simulink model "test_mdl1"  (R2023a)
settings: Solver=VariableStepAuto  StartTime=0.0  StopTime=10.0  RelTol=1e-3
(part 6 of 8)

== system test_mdl1/VehicleCAN/IPMA_ADAS/IPMA_Data3 ==
  AdbUrbanArea_B_Stat : Constant  Value=0
  CbdblActv_B_RqAdas : Constant  Value=0
  LightCurv_NoRate_Actl : Constant  Value=0
  LightCurv_No_Actl : Constant  Value=0
  LightPathOffst_L_Actl : Constant  Value=0
  LightPath_An_Actl : Constant  Value=0
  LightRng_L_Max : Constant  Value=0
  MbdblActv_B_RqAdas : Constant  Value=0
  bus_creator : BusCreator  Inputs=8
  out_port : Outport
  wires:
  bus_creator/1 -> out_port/1  "test_mdl1"
  AdbUrbanArea_B_Stat/1 -> bus_creator/1  "AdbUrbanArea_B_Stat"
  CbdblActv_B_RqAdas/1 -> bus_creator/2  "CbdblActv_B_RqAdas"
  LightCurv_NoRate_Actl/1 -> bus_creator/3  "LightCurv_NoRate_Actl"
  LightCurv_No_Actl/1 -> bus_creator/4  "LightCurv_No_Actl"
  LightPathOffst_L_Actl/1 -> bus_creator/5  "LightPathOffst_L_Actl"
  LightPath_An_Actl/1 -> bus_creator/6  "LightPath_An_Actl"
  LightRng_L_Max/1 -> bus_creator/7  "LightRng_L_Max"
  MbdblActv_B_RqAdas/1 -> bus_creator/8  "MbdblActv_B_RqAdas"

== system test_mdl1/VehicleCAN/IPMA_ADAS/IPMA_Data4 ==
  AdasLcDistToObj_L_Actl : Constant  Value=0
  VehVActlAdas_D_Qf : Constant  Value=0
  Veh_V_ActlAdas : Constant  Value=0
  Veh_V_RqLsc : Constant  Value=0
  bus_creator : BusCreator  Inputs=4
  out_port : Outport
  wires:
  bus_creator/1 -> out_port/1  "test_mdl1"
  AdasLcDistToObj_L_Actl/1 -> bus_creator/1  "AdasLcDistToObj_L_Actl"
  VehVActlAdas_D_Qf/1 -> bus_creator/2  "VehVActlAdas_D_Qf"
  Veh_V_ActlAdas/1 -> bus_creator/3  "Veh_V_ActlAdas"
  Veh_V_RqLsc/1 -> bus_creator/4  "Veh_V_RqLsc"

== system test_mdl1/VehicleCAN/IPMA_ADAS/Image_Processing_Data ==
  BrkDecel_B_RqRba : Constant  Value=0
  BrkEnbl_B_RqRba : Constant  Value=0
  CamraFrntStat_D_Stat : Constant  Value=0
  RbaAlrt_D_Dsply : Constant  Value=0
  RbaMnu_D_Rq : Constant  Value=0
  RbaMsg_D_Rq : Constant  Value=0
  Rba_D_Stat : Constant  Value=0
  TrlrAidEnbl_D_RqAdas : Constant  Value=0
  TrlrAidSwtchLamp_B_Rq : Constant  Value=0
  TrlrHitchChime_D_Rq : Constant  Value=0
  TrlrHitchIcon_D_Rq : Constant  Value=0
  TrlrHitchLamp_D_Rq2 : Constant  Value=0
  TrlrHitchMsgTxt_D_Rq : Constant  Value=0
  TrlrRvrseEnbl_D2_Stat : Constant  Value=0
  TrlrRvrseMsgTxt_D2_Rq : Constant  Value=0
  bus_creator : BusCreator  Inputs=15
  out_port : Outport
  wires:
  bus_creator/1 -> out_port/1  "test_mdl1"
  BrkDecel_B_RqRba/1 -> bus_creator/1  "BrkDecel_B_RqRba"
  BrkEnbl_B_RqRba/1 -> bus_creator/2  "BrkEnbl_B_RqRba"
  CamraFrntStat_D_Stat/1 -> bus_creator/3  "CamraFrntStat_D_Stat"
  RbaAlrt_D_Dsply/1 -> bus_creator/4  "RbaAlrt_D_Dsply"
  RbaMnu_D_Rq/1 -> bus_creator/5  "RbaMnu_D_Rq"
  RbaMsg_D_Rq/1 -> bus_creator/6  "RbaMsg_D_Rq"
  Rba_D_Stat/1 -> bus_creator/7  "Rba_D_Stat"
  TrlrAidEnbl_D_RqAdas/1 -> bus_creator/8  "TrlrAidEnbl_D_RqAdas"
  TrlrAidSwtchLamp_B_Rq/1 -> bus_creator/9  "TrlrAidSwtchLamp_B_Rq"
  TrlrHitchChime_D_Rq/1 -> bus_creator/10  "TrlrHitchChime_D_Rq"
  TrlrHitchIcon_D_Rq/1 -> bus_creator/11  "TrlrHitchIcon_D_Rq"
  TrlrHitchLamp_D_Rq2/1 -> bus_creator/12  "TrlrHitchLamp_D_Rq2"
  TrlrHitchMsgTxt_D_Rq/1 -> bus_creator/13  "TrlrHitchMsgTxt_D_Rq"
  TrlrRvrseEnbl_D2_Stat/1 -> bus_creator/14  "TrlrRvrseEnbl_D2_Stat"
  TrlrRvrseMsgTxt_D2_Rq/1 -> bus_creator/15  "TrlrRvrseMsgTxt_D2_Rq"

== system test_mdl1/VehicleCAN/IPMA_ADAS/Lane_Assist_Data1 ==
  LaCurvature_No_Calc : Constant  Value=0
  LaRampType_B_Req : Constant  Value=0
  LaRefAng_No_Req : Constant  Value=0
  LdwActvIntns_D_Req : Constant  Value=0
  LdwActvStats_D_Req : Constant  Value=0
  LkaActvStats_D2_Req : Constant  Value=0
  LkaDrvOvrrd_D_Rq : Constant  Value=0
  bus_creator : BusCreator  Inputs=7
  out_port : Outport
  wires:
  bus_creator/1 -> out_port/1  "test_mdl1"
  LaCurvature_No_Calc/1 -> bus_creator/1  "LaCurvature_No_Calc"
  LaRampType_B_Req/1 -> bus_creator/2  "LaRampType_B_Req"
  LaRefAng_No_Req/1 -> bus_creator/3  "LaRefAng_No_Req"
  LdwActvIntns_D_Req/1 -> bus_creator/4  "LdwActvIntns_D_Req"
  LdwActvStats_D_Req/1 -> bus_creator/5  "LdwActvStats_D_Req"
  LkaActvStats_D2_Req/1 -> bus_creator/6  "LkaActvStats_D2_Req"
  LkaDrvOvrrd_D_Rq/1 -> bus_creator/7  "LkaDrvOvrrd_D_Rq"

== system test_mdl1/VehicleCAN/IPMA_ADAS/LateralMotionControl ==
  HandsOffCnfm_B_Rq : Constant  Value=0
  LatCtlCurv_NoRate_Actl : Constant  Value=0
  LatCtlCurv_No_Actl : Constant  Value=0
  LatCtlPathOffst_L_Actl : Constant  Value=0
  LatCtlPath_An_Actl : Constant  Value=0
  LatCtlPrecision_D_Rq : Constant  Value=0
  LatCtlRampType_D_Rq : Constant  Value=0
  LatCtlRng_L_Max : Constant  Value=0
  LatCtl_D_Rq : Constant  Value=0
  bus_creator : BusCreator  Inputs=9
  out_port : Outport
  wires:
  bus_creator/1 -> out_port/1  "test_mdl1"
  HandsOffCnfm_B_Rq/1 -> bus_creator/1  "HandsOffCnfm_B_Rq"
  LatCtlCurv_NoRate_Actl/1 -> bus_creator/2  "LatCtlCurv_NoRate_Actl"
  LatCtlCurv_No_Actl/1 -> bus_creator/3  "LatCtlCurv_No_Actl"
  LatCtlPathOffst_L_Actl/1 -> bus_creator/4  "LatCtlPathOffst_L_Actl"
  LatCtlPath_An_Actl/1 -> bus_creator/5  "LatCtlPath_An_Actl"
  LatCtlPrecision_D_Rq/1 -> bus_creator/6  "LatCtlPrecision_D_Rq"
  LatCtlRampType_D_Rq/1 -> bus_creator/7  "LatCtlRampType_D_Rq"
  LatCtlRng_L_Max/1 -> bus_creator/8  "LatCtlRng_L_Max"
  LatCtl_D_Rq/1 -> bus_creator/9  "LatCtl_D_Rq"

== system test_mdl1/VehicleCAN/IPMA_ADAS/LateralMotionControl2 ==
  HandsOffCnfm_B_Rq : Constant  Value=0
  LatCtlCrv_NoRate2_Actl : Constant  Value=0
  LatCtlCurv_No_Actl : Constant  Value=0
  LatCtlPathOffst_L_Actl : Constant  Value=0
  LatCtlPath_An_Actl : Constant  Value=0
  LatCtlPath_No_Cnt : Constant  Value=0
  LatCtlPath_No_Cs : Constant  Value=0
  LatCtlPrecision_D_Rq : Constant  Value=0
  LatCtlRampType_D_Rq : Constant  Value=0
  LatCtl_D2_Rq : Constant  Value=0
  bus_creator : BusCreator  Inputs=10
  out_port : Outport
  wires:
  bus_creator/1 -> out_port/1  "test_mdl1"
  HandsOffCnfm_B_Rq/1 -> bus_creator/1  "HandsOffCnfm_B_Rq"
  LatCtlCrv_NoRate2_Actl/1 -> bus_creator/2  "LatCtlCrv_NoRate2_Actl"
  LatCtlCurv_No_Actl/1 -> bus_creator/3  "LatCtlCurv_No_Actl"
  LatCtlPathOffst_L_Actl/1 -> bus_creator/4  "LatCtlPathOffst_L_Actl"
  LatCtlPath_An_Actl/1 -> bus_creator/5  "LatCtlPath_An_Actl"
  LatCtlPath_No_Cnt/1 -> bus_creator/6  "LatCtlPath_No_Cnt"
  LatCtlPath_No_Cs/1 -> bus_creator/7  "LatCtlPath_No_Cs"
  LatCtlPrecision_D_Rq/1 -> bus_creator/8  "LatCtlPrecision_D_Rq"
  LatCtlRampType_D_Rq/1 -> bus_creator/9  "LatCtlRampType_D_Rq"
  LatCtl_D2_Rq/1 -> bus_creator/10  "LatCtl_D2_Rq"

== system test_mdl1/VehicleCAN/IPMA_ADAS/OTAPhysCCMtoGWM_ECG ==
  OTAPhysCCMtoGWM_ECG : Constant  Value=0
  bus_creator : BusCreator  Inputs=1
  out_port : Outport
  wires:
  bus_creator/1 -> out_port/1  "test_mdl1"
  OTAPhysCCMtoGWM_ECG/1 -> bus_creator/1  "OTAPhysCCMtoGWM_ECG"

== system test_mdl1/VehicleCAN/IPMA_ADAS/OTAPhysIPMAtoGWM_ECG ==
  OTAPhysIPMAtoGWM_ECG : Constant  Value=0
  bus_creator : BusCreator  Inputs=1
  out_port : Outport
  wires:
  bus_creator/1 -> out_port/1  "test_mdl1"
  OTAPhysIPMAtoGWM_ECG/1 -> bus_creator/1  "OTAPhysIPMAtoGWM_ECG"

== system test_mdl1/VehicleCAN/IPMA_ADAS/OTAPhysSODCMCtoGWM_ECG ==
  OTAPhysSODCMCtoGWM_ECG : Constant  Value=0
  bus_creator : BusCreator  Inputs=1
  out_port : Outport
  wires:
  bus_creator/1 -> out_port/1  "test_mdl1"
  OTAPhysSODCMCtoGWM_ECG/1 -> bus_creator/1  "OTAPhysSODCMCtoGWM_ECG"

== system test_mdl1/VehicleCAN/IPMA_ADAS/OTAPhysSODCMDtoGWM_ECG ==
  OTAPhysSODCMDtoGWM_ECG : Constant  Value=0
  bus_creator : BusCreator  Inputs=1
  out_port : Outport
  wires:
  bus_creator/1 -> out_port/1  "test_mdl1"
  OTAPhysSODCMDtoGWM_ECG/1 -> bus_creator/1  "OTAPhysSODCMDtoGWM_ECG"

== system test_mdl1/VehicleCAN/IPMA_ADAS/OTAPhysSODLtoGWM_ECG ==
  OTAPhysSODLtoGWM_ECG : Constant  Value=0
  bus_creator : BusCreator  Inputs=1
  out_port : Outport
  wires:
  bus_creator/1 -> out_port/1  "test_mdl1"
  OTAPhysSODLtoGWM_ECG/1 -> bus_creator/1  "OTAPhysSODLtoGWM_ECG"

== system test_mdl1/VehicleCAN/IPMA_ADAS/OTAPhysSODRtoGWM_ECG ==
  OTAPhysSODRtoGWM_ECG : Constant  Value=0
  bus_creator : BusCreator  Inputs=1
  out_port : Outport
  wires:
  bus_creator/1 -> out_port/1  "test_mdl1"
  OTAPhysSODRtoGWM_ECG/1 -> bus_creator/1  "OTAPhysSODRtoGWM_ECG"

== system test_mdl1/VehicleCAN/IPMA_ADAS/PARSEDPhysCCMtoGWM_ECG ==
  PARSEDPhysCCMtoGWM_ECG : Constant  Value=0
  bus_creator : BusCreator  Inputs=1
  out_port : Outport
  wires:
  bus_creator/1 -> out_port/1  "test_mdl1"
  PARSEDPhysCCMtoGWM_ECG/1 -> bus_creator/1  "PARSEDPhysCCMtoGWM_ECG"

== system test_mdl1/VehicleCAN/IPMA_ADAS/PARSEDPhysIPMAtoGWM_ECG ==
  PARSEDPhysIPMAtoGWM_ECG : Constant  Value=0
  bus_creator : BusCreator  Inputs=1
  out_port : Outport
  wires:
  bus_creator/1 -> out_port/1  "test_mdl1"
  PARSEDPhysIPMAtoGWM_ECG/1 -> bus_creator/1  "PARSEDPhysIPMAtoGWM_ECG"

== system test_mdl1/VehicleCAN/IPMA_ADAS/PARSEDPhysSODCMCtoGWM_ECG ==
  PARSEDPhysSODCMCtoGWM_ECG : Constant  Value=0
  bus_creator : BusCreator  Inputs=1
  out_port : Outport
  wires:
  bus_creator/1 -> out_port/1  "test_mdl1"
  PARSEDPhysSODCMCtoGWM_ECG/1 -> bus_creator/1  "PARSEDPhysSODCMCtoGWM_ECG"

== system test_mdl1/VehicleCAN/IPMA_ADAS/PARSEDPhysSODCMDtoGWM_ECG ==
  PARSEDPhysSODCMDtoGWM_ECG : Constant  Value=0
  bus_creator : BusCreator  Inputs=1
  out_port : Outport
  wires:
  bus_creator/1 -> out_port/1  "test_mdl1"
  PARSEDPhysSODCMDtoGWM_ECG/1 -> bus_creator/1  "PARSEDPhysSODCMDtoGWM_ECG"

== system test_mdl1/VehicleCAN/IPMA_ADAS/PARSEDPhysSODLtoGWM_ECG ==
  PARSEDPhysSODLtoGWM_ECG : Constant  Value=0
  bus_creator : BusCreator  Inputs=1
  out_port : Outport
  wires:
  bus_creator/1 -> out_port/1  "test_mdl1"
  PARSEDPhysSODLtoGWM_ECG/1 -> bus_creator/1  "PARSEDPhysSODLtoGWM_ECG"

== system test_mdl1/VehicleCAN/IPMA_ADAS/PARSEDPhysSODRtoGWM_ECG ==
  PARSEDPhysSODRtoGWM_ECG : Constant  Value=0
  bus_creator : BusCreator  Inputs=1
  out_port : Outport
  wires:
  bus_creator/1 -> out_port/1  "test_mdl1"
  PARSEDPhysSODRtoGWM_ECG/1 -> bus_creator/1  "PARSEDPhysSODRtoGWM_ECG"

== system test_mdl1/VehicleCAN/IPMA_ADAS/PARSEDPushCCMtoGWM_ECG ==
  PARSEDPhysCCM2toGWM_ECG : Constant  Value=0
  bus_creator : BusCreator  Inputs=1
  out_port : Outport
  wires:
  bus_creator/1 -> out_port/1  "test_mdl1"
  PARSEDPhysCCM2toGWM_ECG/1 -> bus_creator/1  "PARSEDPhysCCM2toGWM_ECG"

== system test_mdl1/VehicleCAN/IPMA_ADAS/PARSEDPushIPMAtoGWM_ECG ==
  PARSEDPhysIPMA2toGWM_ECG : Constant  Value=0
  bus_creator : BusCreator  Inputs=1
  out_port : Outport
  wires:
  bus_creator/1 -> out_port/1  "test_mdl1"
  PARSEDPhysIPMA2toGWM_ECG/1 -> bus_creator/1  "PARSEDPhysIPMA2toGWM_ECG"

== system test_mdl1/VehicleCAN/IPMA_ADAS/PARSEDPushSODCMCtoGWM ==
  PARSEDPhysSODCMC2toGWM_ECG : Constant  Value=0
  bus_creator : BusCreator  Inputs=1
  out_port : Outport
  wires:
  bus_creator/1 -> out_port/1  "test_mdl1"
  PARSEDPhysSODCMC2toGWM_ECG/1 -> bus_creator/1  "PARSEDPhysSODCMC2toGWM_ECG"

== system test_mdl1/VehicleCAN/IPMA_ADAS/PARSEDPushSODCMDtoGWM ==
  PARSEDPhysSODCMD2toGWM_ECG : Constant  Value=0
  bus_creator : BusCreator  Inputs=1
  out_port : Outport
  wires:
  bus_creator/1 -> out_port/1  "test_mdl1"
  PARSEDPhysSODCMD2toGWM_ECG/1 -> bus_creator/1  "PARSEDPhysSODCMD2toGWM_ECG"

== system test_mdl1/VehicleCAN/IPMA_ADAS/PARSEDPushSODLtoGWM_ECG ==
  PARSEDPhysSODL2toGWM_ECG : Constant  Value=0
  bus_creator : BusCreator  Inputs=1
  out_port : Outport
  wires:
  bus_creator/1 -> out_port/1  "test_mdl1"
  PARSEDPhysSODL2toGWM_ECG/1 -> bus_creator/1  "PARSEDPhysSODL2toGWM_ECG"

== system test_mdl1/VehicleCAN/IPMA_ADAS/PARSEDPushSODRtoGWM_ECG ==
  PARSEDPhysSODR2toGWM_ECG : Constant  Value=0
  bus_creator : BusCreator  Inputs=1
  out_port : Outport
  wires:
  bus_creator/1 -> out_port/1  "test_mdl1"
  PARSEDPhysSODR2toGWM_ECG/1 -> bus_creator/1  "PARSEDPhysSODR2toGWM_ECG"

== system test_mdl1/VehicleCAN/IPMA_ADAS/ParkAid_Aud_Warn_Stat ==
  ApaActvSd_D_Actl : Constant  Value=0
  ApaMde_D_Avail : Constant  Value=0
  ApaMde_D_Stat : Constant  Value=0
  FpaChime_D_Rq : Constant  Value=0
  PrkAidAudioMute_B_Rq : Constant  Value=0
  PrkAidMsgTxt_D_Rq : Constant  Value=0
  PrkAidSnsFlCntr_D_Stat : Constant  Value=0
  PrkAidSnsFlCrnr_D_Stat : Constant  Value=0
  PrkAidSnsFrCntr_D_Stat : Constant  Value=0
  PrkAidSnsFrCrnr_D_Stat : Constant  Value=0
  PrkAidSwtch_B_Stat : Constant  Value=0
  PrkBrkEl_B_RqFap : Constant  Value=0
  RpaChime_D_Rq : Constant  Value=0
  SidePrkSnsL1_D_Stat : Constant  Value=0
  SidePrkSnsL2_D_Stat : Constant  Value=0
  SidePrkSnsR1_D_Stat : Constant  Value=0
  SidePrkSnsR2_D_Stat : Constant  Value=0
  bus_creator : BusCreator  Inputs=17
  out_port : Outport
  wires:
  bus_creator/1 -> out_port/1  "test_mdl1"
  ApaActvSd_D_Actl/1 -> bus_creator/1  "ApaActvSd_D_Actl"
  ApaMde_D_Avail/1 -> bus_creator/2  "ApaMde_D_Avail"
  ApaMde_D_Stat/1 -> bus_creator/3  "ApaMde_D_Stat"
  FpaChime_D_Rq/1 -> bus_creator/4  "FpaChime_D_Rq"
  PrkAidAudioMute_B_Rq/1 -> bus_creator/5  "PrkAidAudioMute_B_Rq"
  PrkAidMsgTxt_D_Rq/1 -> bus_creator/6  "PrkAidMsgTxt_D_Rq"
  PrkAidSnsFlCntr_D_Stat/1 -> bus_creator/7  "PrkAidSnsFlCntr_D_Stat"
  PrkAidSnsFlCrnr_D_Stat/1 -> bus_creator/8  "PrkAidSnsFlCrnr_D_Stat"
  PrkAidSnsFrCntr_D_Stat/1 -> bus_creator/9  "PrkAidSnsFrCntr_D_Stat"
  PrkAidSnsFrCrnr_D_Stat/1 -> bus_creator/10  "PrkAidSnsFrCrnr_D_Stat"
  PrkAidSwtch_B_Stat/1 -> bus_creator/11  "PrkAidSwtch_B_Stat"
  PrkBrkEl_B_RqFap/1 -> bus_creator/12  "PrkBrkEl_B_RqFap"
  RpaChime_D_Rq/1 -> bus_creator/13  "RpaChime_D_Rq"
  SidePrkSnsL1_D_Stat/1 -> bus_creator/14  "SidePrkSnsL1_D_Stat"
  SidePrkSnsL2_D_Stat/1 -> bus_creator/15  "SidePrkSnsL2_D_Stat"
  SidePrkSnsR1_D_Stat/1 -> bus_creator/16  "SidePrkSnsR1_D_Stat"
  SidePrkSnsR2_D_Stat/1 -> bus_creator/17  "SidePrkSnsR2_D_Stat"

== system test_mdl1/VehicleCAN/IPMA_ADAS/ParkAid_Aud_Warn_Stat2 ==
  ApaBrk_A_Rq : Constant  Value=0
  ApaBrk_D_Rq : Constant  Value=0
  ApaLongCtrlEnbl_D_Rq : Constant  Value=0
  PrkAidChime_D_Stat : Constant  Value=0
  PrkAidFront_D_Stat : Constant  Value=0
  PrkAidLamp_D_Rq : Constant  Value=0
  PrkAidRear_D_Stat : Constant  Value=0
  PrkAidSnsRlCntr_D_Stat : Constant  Value=0
  PrkAidSnsRlCrnr_D_Stat : Constant  Value=0
  PrkAidSnsRrCntr_D_Stat : Constant  Value=0
  PrkAidSnsRrCrnr_D_Stat : Constant  Value=0
  PrkAid_D_Falt : Constant  Value=0
  SidePrkSnsL3_D_Stat : Constant  Value=0
  SidePrkSnsL4_D_Stat : Constant  Value=0
  SidePrkSnsR3_D_Stat : Constant  Value=0
  SidePrkSnsR4_D_Stat : Constant  Value=0
  bus_creator : BusCreator  Inputs=16
  out_port : Outport
  wires:
  bus_creator/1 -> out_port/1  "test_mdl1"
  ApaBrk_A_Rq/1 -> bus_creator/1  "ApaBrk_A_Rq"
  ApaBrk_D_Rq/1 -> bus_creator/2  "ApaBrk_D_Rq"
  ApaLongCtrlEnbl_D_Rq/1 -> bus_creator/3  "ApaLongCtrlEnbl_D_Rq"
  PrkAidChime_D_Stat/1 -> bus_creator/4  "PrkAidChime_D_Stat"
  PrkAidFront_D_Stat/1 -> bus_creator/5  "PrkAidFront_D_Stat"
  PrkAidLamp_D_Rq/1 -> bus_creator/6  "PrkAidLamp_D_Rq"
  PrkAidRear_D_Stat/1 -> bus_creator/7  "PrkAidRear_D_Stat"
  PrkAidSnsRlCntr_D_Stat/1 -> bus_creator/8  "PrkAidSnsRlCntr_D_Stat"
  PrkAidSnsRlCrnr_D_Stat/1 -> bus_creator/9  "PrkAidSnsRlCrnr_D_Stat"
  PrkAidSnsRrCntr_D_Stat/1 -> bus_creator/10  "PrkAidSnsRrCntr_D_Stat"
  PrkAidSnsRrCrnr_D_Stat/1 -> bus_creator/11  "PrkAidSnsRrCrnr_D_Stat"
  PrkAid_D_Falt/1 -> bus_creator/12  "PrkAid_D_Falt"
  SidePrkSnsL3_D_Stat/1 -> bus_creator/13  "SidePrkSnsL3_D_Stat"
  SidePrkSnsL4_D_Stat/1 -> bus_creator/14  "SidePrkSnsL4_D_Stat"
  SidePrkSnsR3_D_Stat/1 -> bus_creator/15  "SidePrkSnsR3_D_Stat"
  SidePrkSnsR4_D_Stat/1 -> bus_creator/16  "SidePrkSnsR4_D_Stat"

== system test_mdl1/VehicleCAN/IPMA_ADAS/ParkAid_Data ==
  ApaAcsy_D_RqDrv : Constant  Value=0
  ApaActvSide2_D_Stat : Constant  Value=0
  ApaButtnPrssd_B_Stat : Constant  Value=0
  ApaChime_D_Rq : Constant  Value=0
  ApaGearShif_D_RqDrv : Constant  Value=0
  ApaLongCtl_D_RqDrv : Constant  Value=0
  ApaMsgTxt_D_Rq : Constant  Value=0
  ApaScan_D_Stat : Constant  Value=0
  ApaSelPoa_D_Stat : Constant  Value=0
  ApaSelPpa_D_Stat : Constant  Value=0
  ApaSelSapp_D_Stat : Constant  Value=0
  ApaSteScanMde_D_Stat : Constant  Value=0
  ApaSteWhl_D_RqDrv : Constant  Value=0
  ApaSys_D_Stat : Constant  Value=0
  ApaTrgtDist_D_Stat : Constant  Value=0
  EPASExtAngleStatReq : Constant  Value=0
  ExtSteeringAngleReq2 : Constant  Value=0
  SAPPStatusCoding : Constant  Value=0
  bus_creator : BusCreator  Inputs=18
  out_port : Outport
  wires:
  bus_creator/1 -> out_port/1  "test_mdl1"
  ApaAcsy_D_RqDrv/1 -> bus_creator/1  "ApaAcsy_D_RqDrv"
  ApaActvSide2_D_Stat/1 -> bus_creator/2  "ApaActvSide2_D_Stat"
  ApaButtnPrssd_B_Stat/1 -> bus_creator/3  "ApaButtnPrssd_B_Stat"
  ApaChime_D_Rq/1 -> bus_creator/4  "ApaChime_D_Rq"
  ApaGearShif_D_RqDrv/1 -> bus_creator/5  "ApaGearShif_D_RqDrv"
  ApaLongCtl_D_RqDrv/1 -> bus_creator/6  "ApaLongCtl_D_RqDrv"
  ApaMsgTxt_D_Rq/1 -> bus_creator/7  "ApaMsgTxt_D_Rq"
  ApaScan_D_Stat/1 -> bus_creator/8  "ApaScan_D_Stat"
  ApaSelPoa_D_Stat/1 -> bus_creator/9  "ApaSelPoa_D_Stat"
  ApaSelPpa_D_Stat/1 -> bus_creator/10  "ApaSelPpa_D_Stat"
  ApaSelSapp_D_Stat/1 -> bus_creator/11  "ApaSelSapp_D_Stat"
  ApaSteScanMde_D_Stat/1 -> bus_creator/12  "ApaSteScanMde_D_Stat"
  ApaSteWhl_D_RqDrv/1 -> bus_creator/13  "ApaSteWhl_D_RqDrv"
  ApaSys_D_Stat/1 -> bus_creator/14  "ApaSys_D_Stat"
  ApaTrgtDist_D_Stat/1 -> bus_creator/15  "ApaTrgtDist_D_Stat"
  EPASExtAngleStatReq/1 -> bus_creator/16  "EPASExtAngleStatReq"
  ExtSteeringAngleReq2/1 -> bus_creator/17  "ExtSteeringAngleReq2"
  SAPPStatusCoding/1 -> bus_creator/18  "SAPPStatusCoding"

== system test_mdl1/VehicleCAN/IPMA_ADAS/ParkAid_Data2 ==
  PrkAidAcsyFront_D_Stat : Constant  Value=0
  PrkAidAcsyRear_D_Stat : Constant  Value=0
  PrkAidDrvDir_D_Stat : Constant  Value=0
  PrkAidRdiusLeft_L_Dsply : Constant  Value=0
  PrkAidRdiusRight_L_Dsply : Constant  Value=0
  bus_creator : BusCreator  Inputs=5
  out_port : Outport
  wires:
  bus_creator/1 -> out_port/1  "test_mdl1"
  PrkAidAcsyFront_D_Stat/1 -> bus_creator/1  "PrkAidAcsyFront_D_Stat"
  PrkAidAcsyRear_D_Stat/1 -> bus_creator/2  "PrkAidAcsyRear_D_Stat"
  PrkAidDrvDir_D_Stat/1 -> bus_creator/3  "PrkAidDrvDir_D_Stat"
  PrkAidRdiusLeft_L_Dsply/1 -> bus_creator/4  "PrkAidRdiusLeft_L_Dsply"
  PrkAidRdiusRight_L_Dsply/1 -> bus_creator/5  "PrkAidRdiusRight_L_Dsply"

== system test_mdl1/VehicleCAN/IPMA_ADAS/ParkAid_Data_2 ==
  FapLcDistToObj_L_Actl : Constant  Value=0
  TrnRngDRqFap_No_Cnt : Constant  Value=0
  TrnRngDRqFap_No_Cs : Constant  Value=0
  TrnRng_D_RqFap : Constant  Value=0
  Veh_V_RqFap : Constant  Value=0
  bus_creator : BusCreator  Inputs=5
  out_port : Outport
  wires:
  bus_creator/1 -> out_port/1  "test_mdl1"
  FapLcDistToObj_L_Actl/1 -> bus_creator/1  "FapLcDistToObj_L_Actl"
  TrnRngDRqFap_No_Cnt/1 -> bus_creator/2  "TrnRngDRqFap_No_Cnt"
  TrnRngDRqFap_No_Cs/1 -> bus_creator/3  "TrnRngDRqFap_No_Cs"
  TrnRng_D_RqFap/1 -> bus_creator/4  "TrnRng_D_RqFap"
  Veh_V_RqFap/1 -> bus_creator/5  "Veh_V_RqFap"

== system test_mdl1/VehicleCAN/IPMA_ADAS/Side_Detect_L_Stat ==
  BttLeft_D_RqDrv : Constant  Value=0
  BttLeft_D_Stat : Constant  Value=0
  CtaAlrtLeft2_D_Stat : Constant  Value=0
  CtaAlrtLeft_D_Stat : Constant  Value=0
  CtaBrkLeftMsgTxt_B_Rq : Constant  Value=0
  CtaLeftBrkDecel_B_Rq : Constant  Value=0
  CtaLeftBrkEnbl_B_Rq : Constant  Value=0
  CtaLeft_D_Stat : Constant  Value=0
  CtaSnsLeft_D_Stat : Constant  Value=0
  Side_Detect_L_Illum : Constant  Value=0
  SodAlrtLeft_D_Stat : Constant  Value=0
  SodDetctLeft_D_Stat : Constant  Value=0
  SodLeft_D_Stat : Constant  Value=0
  SodSnsLeft_D_Stat : Constant  Value=0
  SodWarnLeft_Prd_Rq : Constant  Value=0
  bus_creator : BusCreator  Inputs=15
  out_port : Outport
  wires:
  bus_creator/1 -> out_port/1  "test_mdl1"
  BttLeft_D_RqDrv/1 -> bus_creator/1  "BttLeft_D_RqDrv"
  BttLeft_D_Stat/1 -> bus_creator/2  "BttLeft_D_Stat"
  CtaAlrtLeft2_D_Stat/1 -> bus_creator/3  "CtaAlrtLeft2_D_Stat"
  CtaAlrtLeft_D_Stat/1 -> bus_creator/4  "CtaAlrtLeft_D_Stat"
  CtaBrkLeftMsgTxt_B_Rq/1 -> bus_creator/5  "CtaBrkLeftMsgTxt_B_Rq"
  CtaLeftBrkDecel_B_Rq/1 -> bus_creator/6  "CtaLeftBrkDecel_B_Rq"
  CtaLeftBrkEnbl_B_Rq/1 -> bus_creator/7  "CtaLeftBrkEnbl_B_Rq"
  CtaLeft_D_Stat/1 -> bus_creator/8  "CtaLeft_D_Stat"
  CtaSnsLeft_D_Stat/1 -> bus_creator/9  "CtaSnsLeft_D_Stat"
  Side_Detect_L_Illum/1 -> bus_creator/10  "Side_Detect_L_Illum"
  SodAlrtLeft_D_Stat/1 -> bus_creator/11  "SodAlrtLeft_D_Stat"
  SodDetctLeft_D_Stat/1 -> bus_creator/12  "SodDetctLeft_D_Stat"
  SodLeft_D_Stat/1 -> bus_creator/13  "SodLeft_D_Stat"
  SodSnsLeft_D_Stat/1 -> bus_creator/14  "SodSnsLeft_D_Stat"
  SodWarnLeft_Prd_Rq/1 -> bus_creator/15  "SodWarnLeft_Prd_Rq"

== system test_mdl1/VehicleCAN/IPMA_ADAS/Side_Detect_R_Stat ==
  BttRight_D_RqDrv : Constant  Value=0
  BttRight_D_Stat : Constant  Value=0
  CtaAlrtRight2_D_Stat : Constant  Value=0
  CtaAlrtRight_D_Stat : Constant  Value=0
  CtaBrkRightMsgTxt_B_Rq : Constant  Value=0
  CtaRightBrkDecel_B_Rq : Constant  Value=0
  CtaRightBrkEnbl_B_Rq : Constant  Value=0
  CtaRight_D_Stat : Constant  Value=0
  CtaSnsRight_D_Stat : Constant  Value=0
  Side_Detect_R_Illum : Constant  Value=0
  SodAlrtRight_D_Stat : Constant  Value=0
  SodDetctRight_D_Stat : Constant  Value=0
  SodRight_D_Stat : Constant  Value=0
  SodSnsRight_D_Stat : Constant  Value=0
  SodWarnRight_Prd_Rq : Constant  Value=0
  bus_creator : BusCreator  Inputs=15
  out_port : Outport
  wires:
  bus_creator/1 -> out_port/1  "test_mdl1"
  BttRight_D_RqDrv/1 -> bus_creator/1  "BttRight_D_RqDrv"
  BttRight_D_Stat/1 -> bus_creator/2  "BttRight_D_Stat"
  CtaAlrtRight2_D_Stat/1 -> bus_creator/3  "CtaAlrtRight2_D_Stat"
  CtaAlrtRight_D_Stat/1 -> bus_creator/4  "CtaAlrtRight_D_Stat"
  CtaBrkRightMsgTxt_B_Rq/1 -> bus_creator/5  "CtaBrkRightMsgTxt_B_Rq"
  CtaRightBrkDecel_B_Rq/1 -> bus_creator/6  "CtaRightBrkDecel_B_Rq"
  CtaRightBrkEnbl_B_Rq/1 -> bus_creator/7  "CtaRightBrkEnbl_B_Rq"
  CtaRight_D_Stat/1 -> bus_creator/8  "CtaRight_D_Stat"
  CtaSnsRight_D_Stat/1 -> bus_creator/9  "CtaSnsRight_D_Stat"
  Side_Detect_R_Illum/1 -> bus_creator/10  "Side_Detect_R_Illum"
  SodAlrtRight_D_Stat/1 -> bus_creator/11  "SodAlrtRight_D_Stat"
  SodDetctRight_D_Stat/1 -> bus_creator/12  "SodDetctRight_D_Stat"
  SodRight_D_Stat/1 -> bus_creator/13  "SodRight_D_Stat"
  SodSnsRight_D_Stat/1 -> bus_creator/14  "SodSnsRight_D_Stat"
  SodWarnRight_Prd_Rq/1 -> bus_creator/15  "SodWarnRight_Prd_Rq"

== system test_mdl1/VehicleCAN/IPMA_ADAS/Steer_Assist_Data ==
  CmbbObjClass_D_Stat : Constant  Value=0
  CmbbObjColl_T_Actl : Constant  Value=0
  CmbbObjConfdnc_D_Stat : Constant  Value=0
  CmbbObjDistLat_L_Actl : Constant  Value=0
  CmbbObjDistLong_L_Actl : Constant  Value=0
  CmbbObjRelLat_V_Actl : Constant  Value=0
  CmbbObjRelLong_V_Actl : Constant  Value=0
  EsaEnbl_D2_Rq : Constant  Value=0
  bus_creator : BusCreator  Inputs=8
  out_port : Outport
  wires:
  bus_creator/1 -> out_port/1  "test_mdl1"
  CmbbObjClass_D_Stat/1 -> bus_creator/1  "CmbbObjClass_D_Stat"
  CmbbObjColl_T_Actl/1 -> bus_creator/2  "CmbbObjColl_T_Actl"
  CmbbObjConfdnc_D_Stat/1 -> bus_creator/3  "CmbbObjConfdnc_D_Stat"
  CmbbObjDistLat_L_Actl/1 -> bus_creator/4  "CmbbObjDistLat_L_Actl"
  CmbbObjDistLong_L_Actl/1 -> bus_creator/5  "CmbbObjDistLong_L_Actl"
  CmbbObjRelLat_V_Actl/1 -> bus_creator/6  "CmbbObjRelLat_V_Actl"
  CmbbObjRelLong_V_Actl/1 -> bus_creator/7  "CmbbObjRelLong_V_Actl"
  EsaEnbl_D2_Rq/1 -> bus_creator/8  "EsaEnbl_D2_Rq"

== system test_mdl1/VehicleCAN/IPMA_ADAS/SuspensionRoad_Data ==
  SrpDistLeft_L_Actl : Constant  Value=0
  SrpDistRight_L_Actl : Constant  Value=0
  SrpEventLeft_D_Stat : Constant  Value=0
  SrpEventRight_D_Stat : Constant  Value=0
  SrpHghtLeft_L_Actl : Constant  Value=0
  SrpHghtRight_L_Actl : Constant  Value=0
  SrpSigValid_B_Stat : Constant  Value=0
  SuspClkSync_No_Actl : Constant  Value=0
  bus_creator : BusCreator  Inputs=8
  out_port : Outport
  wires:
  bus_creator/1 -> out_port/1  "test_mdl1"
  SrpDistLeft_L_Actl/1 -> bus_creator/1  "SrpDistLeft_L_Actl"
  SrpDistRight_L_Actl/1 -> bus_creator/2  "SrpDistRight_L_Actl"
  SrpEventLeft_D_Stat/1 -> bus_creator/3  "SrpEventLeft_D_Stat"
  SrpEventRight_D_Stat/1 -> bus_creator/4  "SrpEventRight_D_Stat"
  SrpHghtLeft_L_Actl/1 -> bus_creator/5  "SrpHghtLeft_L_Actl"
  SrpHghtRight_L_Actl/1 -> bus_creator/6  "SrpHghtRight_L_Actl"
  SrpSigValid_B_Stat/1 -> bus_creator/7  "SrpSigValid_B_Stat"
  SuspClkSync_No_Actl/1 -> bus_creator/8  "SuspClkSync_No_Actl"

== system test_mdl1/VehicleCAN/IPMA_ADAS/TesterPhysicalResCCM ==
  TesterPhysicalResCCM : Constant  Value=0
  bus_creator : BusCreator  Inputs=1
  out_port : Outport
  wires:
  bus_creator/1 -> out_port/1  "test_mdl1"
  TesterPhysicalResCCM/1 -> bus_creator/1  "TesterPhysicalResCCM"

== system test_mdl1/VehicleCAN/IPMA_ADAS/TesterPhysicalResIPMA ==
  TesterPhysicalResIPMA : Constant  Value=0
  bus_creator : BusCreator  Inputs=1
  out_port : Outport
  wires:
  bus_creator/1 -> out_port/1  "test_mdl1"
  TesterPhysicalResIPMA/1 -> bus_creator/1  "TesterPhysicalResIPMA"

== system test_mdl1/VehicleCAN/IPMA_ADAS/TesterPhysicalResSODCMC ==
  TesterPhysicalResSODCMC : Constant  Value=0
  bus_creator : BusCreator  Inputs=1
  out_port : Outport
  wires:
  bus_creator/1 -> out_port/1  "test_mdl1"
  TesterPhysicalResSODCMC/1 -> bus_creator/1  "TesterPhysicalResSODCMC"

== system test_mdl1/VehicleCAN/IPMA_ADAS/TesterPhysicalResSODCMD ==
  TesterPhysicalResSODCMD : Constant  Value=0
  bus_creator : BusCreator  Inputs=1
  out_port : Outport
  wires:
  bus_creator/1 -> out_port/1  "test_mdl1"
  TesterPhysicalResSODCMD/1 -> bus_creator/1  "TesterPhysicalResSODCMD"

== system test_mdl1/VehicleCAN/IPMA_ADAS/TesterPhysicalResSODL ==
  TesterPhysicalResSODL : Constant  Value=0
  bus_creator : BusCreator  Inputs=1
  out_port : Outport
  wires:
  bus_creator/1 -> out_port/1  "test_mdl1"
  TesterPhysicalResSODL/1 -> bus_creator/1  "TesterPhysicalResSODL"

== system test_mdl1/VehicleCAN/IPMA_ADAS/TesterPhysicalResSODR ==
  TesterPhysicalResSODR : Constant  Value=0
  bus_creator : BusCreator  Inputs=1
  out_port : Outport
  wires:
  bus_creator/1 -> out_port/1  "test_mdl1"
  TesterPhysicalResSODR/1 -> bus_creator/1  "TesterPhysicalResSODR"

== system test_mdl1/VehicleCAN/IPMA_ADAS/Traffic_RecognitnData ==
  TsrMsgTxt_D_Rq : Constant  Value=0
  TsrOswWarnMsgTxt_D_Rq : Constant  Value=0
  TsrOvtkMsgTxt2_D_Rq : Constant  Value=0
  TsrOvtkMsgTxt_D_Rq : Constant  Value=0
  TsrOvtkStatMsgTxt_D_Rq : Constant  Value=0
  TsrStatMsgTxt_D_Rq : Constant  Value=0
  TsrVLim1MsgTxt_D_Rq : Constant  Value=0
  TsrVLim2MsgTxt_D_Rq : Constant  Value=0
  TsrVl1PrmntMsgTxt_D_Rq : Constant  Value=0
  TsrVl1RstrcMsgTxt2_D_Rq : Constant  Value=0
  TsrVl1RstrcMsgTxt_D_Rq : Constant  Value=0
  TsrVl1StatMsgTxt_D_Rq : Constant  Value=0
  TsrVl2PrmntMsgTxt_D_Rq : Constant  Value=0
  TsrVl2RstrcMsgTxt2_D_Rq : Constant  Value=0
  TsrVl2RstrcMsgTxt_D_Rq : Constant  Value=0
  TsrVl2StatMsgTxt_D_Rq : Constant  Value=0
  TsrVlUnitMsgTxt_D_Rq : Constant  Value=0
  WwaWarn_B_Rq : Constant  Value=0
  bus_creator : BusCreator  Inputs=18
  out_port : Outport
  wires:
  bus_creator/1 -> out_port/1  "test_mdl1"
  TsrMsgTxt_D_Rq/1 -> bus_creator/1  "TsrMsgTxt_D_Rq"
  TsrOswWarnMsgTxt_D_Rq/1 -> bus_creator/2  "TsrOswWarnMsgTxt_D_Rq"
  TsrOvtkMsgTxt2_D_Rq/1 -> bus_creator/3  "TsrOvtkMsgTxt2_D_Rq"
  TsrOvtkMsgTxt_D_Rq/1 -> bus_creator/4  "TsrOvtkMsgTxt_D_Rq"
  TsrOvtkStatMsgTxt_D_Rq/1 -> bus_creator/5  "TsrOvtkStatMsgTxt_D_Rq"
  TsrStatMsgTxt_D_Rq/1 -> bus_creator/6  "TsrStatMsgTxt_D_Rq"
  TsrVLim1MsgTxt_D_Rq/1 -> bus_creator/7  "TsrVLim1MsgTxt_D_Rq"
  TsrVLim2MsgTxt_D_Rq/1 -> bus_creator/8  "TsrVLim2MsgTxt_D_Rq"
  TsrVl1PrmntMsgTxt_D_Rq/1 -> bus_creator/9  "TsrVl1PrmntMsgTxt_D_Rq"
  TsrVl1RstrcMsgTxt2_D_Rq/1 -> bus_creator/10  "TsrVl1RstrcMsgTxt2_D_Rq"
  TsrVl1RstrcMsgTxt_D_Rq/1 -> bus_creator/11  "TsrVl1RstrcMsgTxt_D_Rq"
  TsrVl1StatMsgTxt_D_Rq/1 -> bus_creator/12  "TsrVl1StatMsgTxt_D_Rq"
  TsrVl2PrmntMsgTxt_D_Rq/1 -> bus_creator/13  "TsrVl2PrmntMsgTxt_D_Rq"
  TsrVl2RstrcMsgTxt2_D_Rq/1 -> bus_creator/14  "TsrVl2RstrcMsgTxt2_D_Rq"
  TsrVl2RstrcMsgTxt_D_Rq/1 -> bus_creator/15  "TsrVl2RstrcMsgTxt_D_Rq"
  TsrVl2StatMsgTxt_D_Rq/1 -> bus_creator/16  "TsrVl2StatMsgTxt_D_Rq"
  TsrVlUnitMsgTxt_D_Rq/1 -> bus_creator/17  "TsrVlUnitMsgTxt_D_Rq"
  WwaWarn_B_Rq/1 -> bus_creator/18  "WwaWarn_B_Rq"

== system test_mdl1/VehicleCAN/IPMA_ADAS/TrailerAid_Stat3 ==
  HitchToTrlrAxle_L_Calc2 : Constant  Value=0
  HitchToVehAxle_L_Calc : Constant  Value=0
  TrlrAidTrgtId_No_Actl : Constant  Value=0
  TrlrAid_An3_Actl : Constant  Value=0
  TrlrAid_AnRate2_Actl : Constant  Value=0
  TrlrAid_D2_Stat : Constant  Value=0
  TrlrAnCalib_B_Complt : Constant  Value=0
  TrlrAnOffstDir_D_Calc : Constant  Value=0
  TrlrAnOffst_An_Calc : Constant  Value=0
  TrlrRvrse_D_Stat : Constant  Value=0
  TrlrTrgtAcquire_D_Stat : Constant  Value=0
  bus_creator : BusCreator  Inputs=11
  out_port : Outport
  wires:
  bus_creator/1 -> out_port/1  "test_mdl1"
  HitchToTrlrAxle_L_Calc2/1 -> bus_creator/1  "HitchToTrlrAxle_L_Calc2"
  HitchToVehAxle_L_Calc/1 -> bus_creator/2  "HitchToVehAxle_L_Calc"
  TrlrAidTrgtId_No_Actl/1 -> bus_creator/3  "TrlrAidTrgtId_No_Actl"
  TrlrAid_An3_Actl/1 -> bus_creator/4  "TrlrAid_An3_Actl"
  TrlrAid_AnRate2_Actl/1 -> bus_creator/5  "TrlrAid_AnRate2_Actl"
  TrlrAid_D2_Stat/1 -> bus_creator/6  "TrlrAid_D2_Stat"
  TrlrAnCalib_B_Complt/1 -> bus_creator/7  "TrlrAnCalib_B_Complt"
  TrlrAnOffstDir_D_Calc/1 -> bus_creator/8  "TrlrAnOffstDir_D_Calc"
  TrlrAnOffst_An_Calc/1 -> bus_creator/9  "TrlrAnOffst_An_Calc"
  TrlrRvrse_D_Stat/1 -> bus_creator/10  "TrlrRvrse_D_Stat"
  TrlrTrgtAcquire_D_Stat/1 -> bus_creator/11  "TrlrTrgtAcquire_D_Stat"

== system test_mdl1/VehicleCAN/PCM/DCACA_Data4 ==
  DcacElPw_D_Stat : Constant  Value=0
  DcacEngOnMsgTxt_D_Rq : Constant  Value=0
  DcacFaltMsgTxt_D_Rq : Constant  Value=0
  DcacGfciTest_B_Rq : Constant  Value=0
  DcacHw_D_Confg : Constant  Value=0
  DcacLedCtl_D_Rq : Constant  Value=0
  DcacLoFuelMsgTxt_D_Rq : Constant  Value=0
  DcacOn_B_Rq : Constant  Value=0
  DcacOut1_Pw_Dsply : Constant  Value=0
  DcacOut2_Pw_Dsply : Constant  Value=0
  DcacOut_Pw_DsplyMx : Constant  Value=0
  DcacSys_B_Falt : Constant  Value=0
  PwBedPnlEnbl_B_Rq : Constant  Value=0
  bus_creator : BusCreator  Inputs=13
  out_port : Outport
  wires:
  bus_creator/1 -> out_port/1  "test_mdl1"
  DcacElPw_D_Stat/1 -> bus_creator/1  "DcacElPw_D_Stat"
  DcacEngOnMsgTxt_D_Rq/1 -> bus_creator/2  "DcacEngOnMsgTxt_D_Rq"
  DcacFaltMsgTxt_D_Rq/1 -> bus_creator/3  "DcacFaltMsgTxt_D_Rq"
  DcacGfciTest_B_Rq/1 -> bus_creator/4  "DcacGfciTest_B_Rq"
  DcacHw_D_Confg/1 -> bus_creator/5  "DcacHw_D_Confg"
  DcacLedCtl_D_Rq/1 -> bus_creator/6  "DcacLedCtl_D_Rq"
  DcacLoFuelMsgTxt_D_Rq/1 -> bus_creator/7  "DcacLoFuelMsgTxt_D_Rq"
  DcacOn_B_Rq/1 -> bus_creator/8  "DcacOn_B_Rq"
  DcacOut1_Pw_Dsply/1 -> bus_creator/9  "DcacOut1_Pw_Dsply"
  DcacOut2_Pw_Dsply/1 -> bus_creator/10  "DcacOut2_Pw_Dsply"
  DcacOut_Pw_DsplyMx/1 -> bus_creator/11  "DcacOut_Pw_DsplyMx"
  DcacSys_B_Falt/1 -> bus_creator/12  "DcacSys_B_Falt"
  PwBedPnlEnbl_B_Rq/1 -> bus_creator/13  "PwBedPnlEnbl_B_Rq"

== system test_mdl1/VehicleCAN/PCM/EngBrakeData ==
  AccEngStat_D_Actl : Constant  Value=0
  AccStopMde_D_Rq : Constant  Value=0
  BPedDrvAppl_D_QF : Constant  Value=0
  BpedDrvAppl_D_Actl : Constant  Value=0
  CcMde_D_Actl : Constant  Value=0
  CcOvrrdActv_B_Actl : Constant  Value=0
  CcStat_D_Actl : Constant  Value=0
  CmbbDeny_B_ActlPrpl : Constant  Value=0
  CmbbEngTqMn_B_Actl : Constant  Value=0
  EngAout_N_MnAllw : Constant  Value=0
  PrplTqMnSat_B_Actl : Constant  Value=0
  Veh_V_DsplyCcSet : Constant  Value=0
  bus_creator : BusCreator  Inputs=12
  out_port : Outport
  wires:
  bus_creator/1 -> out_port/1  "test_mdl1"
  AccEngStat_D_Actl/1 -> bus_creator/1  "AccEngStat_D_Actl"
  AccStopMde_D_Rq/1 -> bus_creator/2  "AccStopMde_D_Rq"
  BPedDrvAppl_D_QF/1 -> bus_creator/3  "BPedDrvAppl_D_QF"
  BpedDrvAppl_D_Actl/1 -> bus_creator/4  "BpedDrvAppl_D_Actl"
  CcMde_D_Actl/1 -> bus_creator/5  "CcMde_D_Actl"
  CcOvrrdActv_B_Actl/1 -> bus_creator/6  "CcOvrrdActv_B_Actl"
  CcStat_D_Actl/1 -> bus_creator/7  "CcStat_D_Actl"
  CmbbDeny_B_ActlPrpl/1 -> bus_creator/8  "CmbbDeny_B_ActlPrpl"
  CmbbEngTqMn_B_Actl/1 -> bus_creator/9  "CmbbEngTqMn_B_Actl"
  EngAout_N_MnAllw/1 -> bus_creator/10  "EngAout_N_MnAllw"
  PrplTqMnSat_B_Actl/1 -> bus_creator/11  "PrplTqMnSat_B_Actl"
  Veh_V_DsplyCcSet/1 -> bus_creator/12  "Veh_V_DsplyCcSet"

== system test_mdl1/VehicleCAN/PCM/EngVehicleSpThrottle ==
  ApedPosPcActl_D_Qf : Constant  Value=0
  ApedPosPcActl_No_Cnt : Constant  Value=0
  ApedPosPcActl_No_Cs : Constant  Value=0
  ApedPos_PcRate_ActlArb : Constant  Value=0
  ApedPos_Pc_ActlArb : Constant  Value=0
  EngAout3_N_Actl : Constant  Value=0
  EngAoutNActl_D_QF : Constant  Value=0
  EngAout_N_Actl : Constant  Value=0
  bus_creator : BusCreator  Inputs=8
  out_port : Outport
  wires:
  bus_creator/1 -> out_port/1  "test_mdl1"
  ApedPosPcActl_D_Qf/1 -> bus_creator/1  "ApedPosPcActl_D_Qf"
  ApedPosPcActl_No_Cnt/1 -> bus_creator/2  "ApedPosPcActl_No_Cnt"
  ApedPosPcActl_No_Cs/1 -> bus_creator/3  "ApedPosPcActl_No_Cs"
  ApedPos_PcRate_ActlArb/1 -> bus_creator/4  "ApedPos_PcRate_ActlArb"
  ApedPos_Pc_ActlArb/1 -> bus_creator/5  "ApedPos_Pc_ActlArb"
  EngAout3_N_Actl/1 -> bus_creator/6  "EngAout3_N_Actl"
  EngAoutNActl_D_QF/1 -> bus_creator/7  "EngAoutNActl_D_QF"
  EngAout_N_Actl/1 -> bus_creator/8  "EngAout_N_Actl"

== system test_mdl1/VehicleCAN/PCM/EngVehicleSpThrottle2 ==
  GearRvrse_D_Actl : Constant  Value=0
  StrtrMtrCtlMsgTxt_D2_Rq : Constant  Value=0
  StrtrMtrCtlMsgTxt_D_Rq : Constant  Value=0
  StrtrMtrDlyStrt_B_Stat : Constant  Value=0
  VehVActlEng_D_Qf : Constant  Value=0
  VehVActlEng_No_Cnt : Constant  Value=0
  VehVActlEng_No_Cs : Constant  Value=0
  VehVTrlrAid_B_Avail : Constant  Value=0
  Veh_V_ActlEng : Constant  Value=0
  Veh_V_RqCcSet : Constant  Value=0
  bus_creator : BusCreator  Inputs=10
  out_port : Outport
  wires:
  bus_creator/1 -> out_port/1  "test_mdl1"
  GearRvrse_D_Actl/1 -> bus_creator/1  "GearRvrse_D_Actl"
  StrtrMtrCtlMsgTxt_D2_Rq/1 -> bus_creator/2  "StrtrMtrCtlMsgTxt_D2_Rq"
  StrtrMtrCtlMsgTxt_D_Rq/1 -> bus_creator/3  "StrtrMtrCtlMsgTxt_D_Rq"
  StrtrMtrDlyStrt_B_Stat/1 -> bus_creator/4  "StrtrMtrDlyStrt_B_Stat"
  VehVActlEng_D_Qf/1 -> bus_creator/5  "VehVActlEng_D_Qf"
  VehVActlEng_No_Cnt/1 -> bus_creator/6  "VehVActlEng_No_Cnt"
  VehVActlEng_No_Cs/1 -> bus_creator/7  "VehVActlEng_No_Cs"
  VehVTrlrAid_B_Avail/1 -> bus_creator/8  "VehVTrlrAid_B_Avail"
  Veh_V_ActlEng/1 -> bus_creator/9  "Veh_V_ActlEng"
  Veh_V_RqCcSet/1 -> bus_creator/10  "Veh_V_RqCcSet"

== system test_mdl1/VehicleCAN/PCM/EngineClimateData ==
  AirAmbTe_D_Qf : Constant  Value=0
  AirAmb_P_Actl : Constant  Value=0
  AirAmb_Te_Actl : Constant  Value=0
  AirAmb_Te_ActlFilt : Constant  Value=0
  AslChime_B_Rq : Constant  Value=0
  AslIconDsply_D_Rq : Constant  Value=0
  DynoMde_B_Cmd : Constant  Value=0
  EcssLamp_D_RqDsply : Constant  Value=0
  EngAout_Aa_Actl : Constant  Value=0
  GasPrtc_D_RqDsply : Constant  Value=0
  HvacHtrCore2_Te_Actl : Constant  Value=0
  bus_creator : BusCreator  Inputs=11
  out_port : Outport
  wires:
  bus_creator/1 -> out_port/1  "test_mdl1"
  AirAmbTe_D_Qf/1 -> bus_creator/1  "AirAmbTe_D_Qf"
  AirAmb_P_Actl/1 -> bus_creator/2  "AirAmb_P_Actl"
  AirAmb_Te_Actl/1 -> bus_creator/3  "AirAmb_Te_Actl"
  AirAmb_Te_ActlFilt/1 -> bus_creator/4  "AirAmb_Te_ActlFilt"
  AslChime_B_Rq/1 -> bus_creator/5  "AslChime_B_Rq"
  AslIconDsply_D_Rq/1 -> bus_creator/6  "AslIconDsply_D_Rq"
  DynoMde_B_Cmd/1 -> bus_creator/7  "DynoMde_B_Cmd"
  EcssLamp_D_RqDsply/1 -> bus_creator/8  "EcssLamp_D_RqDsply"
  EngAout_Aa_Actl/1 -> bus_creator/9  "EngAout_Aa_Actl"
  GasPrtc_D_RqDsply/1 -> bus_creator/10  "GasPrtc_D_RqDsply"
  HvacHtrCore2_Te_Actl/1 -> bus_creator/11  "HvacHtrCore2_Te_Actl"

== system test_mdl1/VehicleCAN/PCM/EngineData_1 ==
  SeatWorkSrfc_B_Falt : Constant  Value=0
  TrnIpcDsplyGear_D_Actl : Constant  Value=0
  TrnIpcDsplyGear_D_Stat : Constant  Value=0
  TrnIpcDsplyMde_D_Actl : Constant  Value=0
  TrnIpcDsplyMde_D_Stat : Constant  Value=0
  TrnIpcDsplyRng2_D_Actl : Constant  Value=0
  TrnIpcDsplyRng_D_Stat : Constant  Value=0
  bus_creator : BusCreator  Inputs=7
  out_port : Outport
  wires:
  bus_creator/1 -> out_port/1  "test_mdl1"
  SeatWorkSrfc_B_Falt/1 -> bus_creator/1  "SeatWorkSrfc_B_Falt"
  TrnIpcDsplyGear_D_Actl/1 -> bus_creator/2  "TrnIpcDsplyGear_D_Actl"
  TrnIpcDsplyGear_D_Stat/1 -> bus_creator/3  "TrnIpcDsplyGear_D_Stat"
  TrnIpcDsplyMde_D_Actl/1 -> bus_creator/4  "TrnIpcDsplyMde_D_Actl"
  TrnIpcDsplyMde_D_Stat/1 -> bus_creator/5  "TrnIpcDsplyMde_D_Stat"
  TrnIpcDsplyRng2_D_Actl/1 -> bus_creator/6  "TrnIpcDsplyRng2_D_Actl"
  TrnIpcDsplyRng_D_Stat/1 -> bus_creator/7  "TrnIpcDsplyRng_D_Stat"

== system test_mdl1/VehicleCAN/PCM/EngineData_16 ==
  EngAout_N_MxAllw : Constant  Value=0
  EngExhBrkAutoLamp_B_Rq : Constant  Value=0
  EngExhBrkMde_D_Actl : Constant  Value=0
  EngExhBrkOnLamp_B_Rq : Constant  Value=0
  EngOilLvlWarn_D_Rq1 : Constant  Value=0
  bus_creator : BusCreator  Inputs=5
  out_port : Outport
  wires:
  bus_creator/1 -> out_port/1  "test_mdl1"
  EngAout_N_MxAllw/1 -> bus_creator/1  "EngAout_N_MxAllw"
  EngExhBrkAutoLamp_B_Rq/1 -> bus_creator/2  "EngExhBrkAutoLamp_B_Rq"
  EngExhBrkMde_D_Actl/1 -> bus_creator/3  "EngExhBrkMde_D_Actl"
  EngExhBrkOnLamp_B_Rq/1 -> bus_creator/4  "EngExhBrkOnLamp_B_Rq"
  EngOilLvlWarn_D_Rq1/1 -> bus_creator/5  "EngOilLvlWarn_D_Rq1"

== system test_mdl1/VehicleCAN/PCM/EngineData_6 ==
  EngClntTe_D_Qf : Constant  Value=0
  EngClnt_Te_Actl : Constant  Value=0
  EngGoutLss_Tq_Est : Constant  Value=0
  EngOil_Te_Actl : Constant  Value=0
  EngOvrhtMitgActv_D_Ind : Constant  Value=0
  bus_creator : BusCreator  Inputs=5
  out_port : Outport
  wires:
  bus_creator/1 -> out_port/1  "test_mdl1"
  EngClntTe_D_Qf/1 -> bus_creator/1  "EngClntTe_D_Qf"
  EngClnt_Te_Actl/1 -> bus_creator/2  "EngClnt_Te_Actl"
  EngGoutLss_Tq_Est/1 -> bus_creator/3  "EngGoutLss_Tq_Est"
  EngOil_Te_Actl/1 -> bus_creator/4  "EngOil_Te_Actl"
  EngOvrhtMitgActv_D_Ind/1 -> bus_creator/5  "EngOvrhtMitgActv_D_Ind"

== system test_mdl1/VehicleCAN/PCM/EngineData_7 ==
  AirCondClutch_B_Stats : Constant  Value=0
  AirCondRec_B_Rq : Constant  Value=0
  EngOilLife_Pc_Actl : Constant  Value=0
  EngSrvcRqd_B_Rq : Constant  Value=0
  FuelFillInlet_B_Dsply : Constant  Value=0
  FuelFilterLamp_B_Dsply : Constant  Value=0
  FuelFlw_Vl_Dsply : Constant  Value=0
  HvacAirFullOut_B_Rq : Constant  Value=0
  OdoCount : Constant  Value=0
  bus_creator : BusCreator  Inputs=9
  out_port : Outport
  wires:
  bus_creator/1 -> out_port/1  "test_mdl1"
  AirCondClutch_B_Stats/1 -> bus_creator/1  "AirCondClutch_B_Stats"
  AirCondRec_B_Rq/1 -> bus_creator/2  "AirCondRec_B_Rq"
  EngOilLife_Pc_Actl/1 -> bus_creator/3  "EngOilLife_Pc_Actl"
  EngSrvcRqd_B_Rq/1 -> bus_creator/4  "EngSrvcRqd_B_Rq"
  FuelFillInlet_B_Dsply/1 -> bus_creator/5  "FuelFillInlet_B_Dsply"
  FuelFilterLamp_B_Dsply/1 -> bus_creator/6  "FuelFilterLamp_B_Dsply"
  FuelFlw_Vl_Dsply/1 -> bus_creator/7  "FuelFlw_Vl_Dsply"
  HvacAirFullOut_B_Rq/1 -> bus_creator/8  "HvacAirFullOut_B_Rq"
  OdoCount/1 -> bus_creator/9  "OdoCount"

== system test_mdl1/VehicleCAN/PCM/Engine_Clutch_Data ==
  CluPdlPosPcMeas_D_Qf : Constant  Value=0
  CluPdlPos_Pc_Meas : Constant  Value=0
  CluPdl_PcRate_Actl : Constant  Value=0
  EngAoutIdl_N_Ntrl : Constant  Value=0
  EngAout_N_Dsply : Constant  Value=0
  bus_creator : BusCreator  Inputs=5
  out_port : Outport
  wires:
  bus_creator/1 -> out_port/1  "test_mdl1"
  CluPdlPosPcMeas_D_Qf/1 -> bus_creator/1  "CluPdlPosPcMeas_D_Qf"
  CluPdlPos_Pc_Meas/1 -> bus_creator/2  "CluPdlPos_Pc_Meas"
  CluPdl_PcRate_Actl/1 -> bus_creator/3  "CluPdl_PcRate_Actl"
  EngAoutIdl_N_Ntrl/1 -> bus_creator/4  "EngAoutIdl_N_Ntrl"
  EngAout_N_Dsply/1 -> bus_creator/5  "EngAout_N_Dsply"

== system test_mdl1/VehicleCAN/PCM/Gear_Shift_by_Wire_3 ==
  GearSelLck_D_Rq : Constant  Value=0
  PrkBrkActv_D_RqTrnGear : Constant  Value=0
  TrnCmdCnt_B_Actl : Constant  Value=0
  TrnCmdState_B_Actl : Constant  Value=0
  TrnDtpCmd_D_Actl : Constant  Value=0
  TrnGearCmd_No_Cnt : Constant  Value=0
  TrnGearCmd_No_Cs : Constant  Value=0
  TrnGearCmd_Pc_ActlPt : Constant  Value=0
  TrnGearMsgTxt_D_Rq : Constant  Value=0
  TrnGearNtmAllow_B_Stat : Constant  Value=0
  TrnGear_D_RqPt : Constant  Value=0
  TrnLvrV_D_Rq : Constant  Value=0
  TrnNtrlTowCmd_D_Actl : Constant  Value=0
  TrnSbwSysHlth_D_Actl : Constant  Value=0
  TrnValidGear_D_Cnfm : Constant  Value=0
  bus_creator : BusCreator  Inputs=15
  out_port : Outport
  wires:
  bus_creator/1 -> out_port/1  "test_mdl1"
  GearSelLck_D_Rq/1 -> bus_creator/1  "GearSelLck_D_Rq"
  PrkBrkActv_D_RqTrnGear/1 -> bus_creator/2  "PrkBrkActv_D_RqTrnGear"
  TrnCmdCnt_B_Actl/1 -> bus_creator/3  "TrnCmdCnt_B_Actl"
  TrnCmdState_B_Actl/1 -> bus_creator/4  "TrnCmdState_B_Actl"
  TrnDtpCmd_D_Actl/1 -> bus_creator/5  "TrnDtpCmd_D_Actl"
  TrnGearCmd_No_Cnt/1 -> bus_creator/6  "TrnGearCmd_No_Cnt"
  TrnGearCmd_No_Cs/1 -> bus_creator/7  "TrnGearCmd_No_Cs"
  TrnGearCmd_Pc_ActlPt/1 -> bus_creator/8  "TrnGearCmd_Pc_ActlPt"
  TrnGearMsgTxt_D_Rq/1 -> bus_creator/9  "TrnGearMsgTxt_D_Rq"
  TrnGearNtmAllow_B_Stat/1 -> bus_creator/10  "TrnGearNtmAllow_B_Stat"
  TrnGear_D_RqPt/1 -> bus_creator/11  "TrnGear_D_RqPt"
  TrnLvrV_D_Rq/1 -> bus_creator/12  "TrnLvrV_D_Rq"
  TrnNtrlTowCmd_D_Actl/1 -> bus_creator/13  "TrnNtrlTowCmd_D_Actl"
  TrnSbwSysHlth_D_Actl/1 -> bus_creator/14  "TrnSbwSysHlth_D_Actl"
  TrnValidGear_D_Cnfm/1 -> bus_creator/15  "TrnValidGear_D_Cnfm"

== system test_mdl1/VehicleCAN/PCM/Global_PATS_TargetInfo ==
  bus_creator : BusCreator  Inputs=3
  immoTarget1Cmd : Constant  Value=0
  immoTarget1Data : Constant  Value=0
  immoTarget1Status : Constant  Value=0
  out_port : Outport
  wires:
  bus_creator/1 -> out_port/1  "test_mdl1"
  immoTarget1Cmd/1 -> bus_creator/1  "immoTarget1Cmd"
  immoTarget1Data/1 -> bus_creator/2  "immoTarget1Data"
  immoTarget1Status/1 -> bus_creator/3  "immoTarget1Status"

== system test_mdl1/VehicleCAN/PCM/Low_Voltage_Power_Data_FD1 ==
  PwSrcULoComm_B_Falt : Constant  Value=0
  PwSrcULoDcnnt_B_Stat : Constant  Value=0
  PwSrcULoFalt_D_Stat : Constant  Value=0
  PwSrcULoOvrTe_B_Actl : Constant  Value=0
  PwSrcULo_I_Actl : Constant  Value=0
  PwSrcULo_I_Mx : Constant  Value=0
  PwSrcULo_Pc_Mx : Constant  Value=0
  ULoRgenTestMde_B_Stat : Constant  Value=0
  bus_creator : BusCreator  Inputs=8
  out_port : Outport
  wires:
  bus_creator/1 -> out_port/1  "test_mdl1"
  PwSrcULoComm_B_Falt/1 -> bus_creator/1  "PwSrcULoComm_B_Falt"
  PwSrcULoDcnnt_B_Stat/1 -> bus_creator/2  "PwSrcULoDcnnt_B_Stat"
  PwSrcULoFalt_D_Stat/1 -> bus_creator/3  "PwSrcULoFalt_D_Stat"
  PwSrcULoOvrTe_B_Actl/1 -> bus_creator/4  "PwSrcULoOvrTe_B_Actl"
  PwSrcULo_I_Actl/1 -> bus_creator/5  "PwSrcULo_I_Actl"
  PwSrcULo_I_Mx/1 -> bus_creator/6  "PwSrcULo_I_Mx"
  PwSrcULo_Pc_Mx/1 -> bus_creator/7  "PwSrcULo_Pc_Mx"
  ULoRgenTestMde_B_Stat/1 -> bus_creator/8  "ULoRgenTestMde_B_Stat"

== system test_mdl1/VehicleCAN/PCM/OTAPhysPCMtoGWM_ECG ==
  OTAPhysPCMtoGWM_ECG : Constant  Value=0
  bus_creator : BusCreator  Inputs=1
  out_port : Outport
  wires:
  bus_creator/1 -> out_port/1  "test_mdl1"
  OTAPhysPCMtoGWM_ECG/1 -> bus_creator/1  "OTAPhysPCMtoGWM_ECG"

== system test_mdl1/VehicleCAN/PCM/PARSEDPhysPCMtoGWM_ECG ==
  PARSEDPhysPCMtoGWM_ECG : Constant  Value=0
  bus_creator : BusCreator  Inputs=1
  out_port : Outport
  wires:
  bus_creator/1 -> out_port/1  "test_mdl1"
  PARSEDPhysPCMtoGWM_ECG/1 -> bus_creator/1  "PARSEDPhysPCMtoGWM_ECG"

== system test_mdl1/VehicleCAN/PCM/PARSEDPushPCMtoGWM_ECG ==
  PARSEDPushPCMtoGWM_ECG : Constant  Value=0
  bus_creator : BusCreator  Inputs=1
  out_port : Outport
  wires:
  bus_creator/1 -> out_port/1  "test_mdl1"
  PARSEDPushPCMtoGWM_ECG/1 -> bus_creator/1  "PARSEDPushPCMtoGWM_ECG"

== system test_mdl1/VehicleCAN/PCM/PCM_AutoSar_NetworkMgmt ==
  PCM_AutoSarNMControl : Constant  Value=0
  PCM_AutoSarNMNodeId : Constant  Value=0
  PCM_AutoSarNMReserved{1..4} (4 alike) : Constant  Value=0
  PCM_GWNMProxy : Constant  Value=0
  PCM_GWOnBoardTester : Constant  Value=0
  bus_creator : BusCreator  Inputs=8
  out_port : Outport
  wires:
  bus_creator/1 -> out_port/1  "test_mdl1"
  PCM_AutoSarNMControl/1 -> bus_creator/1  "PCM_AutoSarNMControl"
  PCM_AutoSarNMNodeId/1 -> bus_creator/2  "PCM_AutoSarNMNodeId"
  PCM_AutoSarNMReserved1/1 -> bus_creator/3  "PCM_AutoSarNMReserved1"
  PCM_AutoSarNMReserved2/1 -> bus_creator/4  "PCM_AutoSarNMReserved2"
  PCM_AutoSarNMReserved3/1 -> bus_creator/5  "PCM_AutoSarNMReserved3"
  PCM_AutoSarNMReserved4/1 -> bus_creator/6  "PCM_AutoSarNMReserved4"
  PCM_GWNMProxy/1 -> bus_creator/7  "PCM_GWNMProxy"
  PCM_GWOnBoardTester/1 -> bus_creator/8  "PCM_GWOnBoardTester"

== system test_mdl1/VehicleCAN/PCM/PCM_Rapid_Data_Response_1 ==
  UUDTPCMResponse1 : Constant  Value=0
  bus_creator : BusCreator  Inputs=1
  out_port : Outport
  wires:
  bus_creator/1 -> out_port/1  "test_mdl1"
  UUDTPCMResponse1/1 -> bus_creator/1  "UUDTPCMResponse1"

== system test_mdl1/VehicleCAN/PCM/PCM_Rapid_Data_Response_2 ==
  UUDTPCMResponse2 : Constant  Value=0
  bus_creator : BusCreator  Inputs=1
  out_port : Outport
  wires:
  bus_creator/1 -> out_port/1  "test_mdl1"
  UUDTPCMResponse2/1 -> bus_creator/1  "UUDTPCMResponse2"

== system test_mdl1/VehicleCAN/PCM/PowertrainData_1 ==
  AirCondFluidHi_P_Actl : Constant  Value=0
  CoolantFanStepAct : Constant  Value=0
  ECMMILRequest : Constant  Value=0
  EngIdlShutDown_D_Stat : Constant  Value=0
  EngIdlShutDwnTxt_D_Rq : Constant  Value=0
  FUEL_ALCOHOL_PERCNT : Constant  Value=0
  FohEng_D_Rq : Constant  Value=0
  OilPressureWarning : Constant  Value=0
  TrnTotLss_Tq_Est : Constant  Value=0
  TrnTotTq_Rt_Est : Constant  Value=0
  VehVLimActv_B_Actl : Constant  Value=0
  VehVLimStat_D_Actl : Constant  Value=0
  bus_creator : BusCreator  Inputs=12
  out_port : Outport
  wires:
  bus_creator/1 -> out_port/1  "test_mdl1"
  AirCondFluidHi_P_Actl/1 -> bus_creator/1  "AirCondFluidHi_P_Actl"
  CoolantFanStepAct/1 -> bus_creator/2  "CoolantFanStepAct"
  ECMMILRequest/1 -> bus_creator/3  "ECMMILRequest"
  EngIdlShutDown_D_Stat/1 -> bus_creator/4  "EngIdlShutDown_D_Stat"
  EngIdlShutDwnTxt_D_Rq/1 -> bus_creator/5  "EngIdlShutDwnTxt_D_Rq"
  FUEL_ALCOHOL_PERCNT/1 -> bus_creator/6  "FUEL_ALCOHOL_PERCNT"
  FohEng_D_Rq/1 -> bus_creator/7  "FohEng_D_Rq"
  OilPressureWarning/1 -> bus_creator/8  "OilPressureWarning"
  TrnTotLss_Tq_Est/1 -> bus_creator/9  "TrnTotLss_Tq_Est"
  TrnTotTq_Rt_Est/1 -> bus_creator/10  "TrnTotTq_Rt_Est"
  VehVLimActv_B_Actl/1 -> bus_creator/11  "VehVLimActv_B_Actl"
  VehVLimStat_D_Actl/1 -> bus_creator/12  "VehVLimStat_D_Actl"

== system test_mdl1/VehicleCAN/PCM/PowertrainData_10 ==
  GearEngag_D_Actl : Constant  Value=0
  GearLvr_D_ActlDrv : Constant  Value=0
  GearPos_D_Actl : Constant  Value=0
  GearPos_D_Trg : Constant  Value=0
  GearPos_No_Cnt : Constant  Value=0
  GearPos_No_Cs : Constant  Value=0
  TrnIgnOffDly_T_Rq : Constant  Value=0
  TrnPrkSys_D_Actl : Constant  Value=0
  TrnRng_D_Rq : Constant  Value=0
  bus_creator : BusCreator  Inputs=9
  out_port : Outport
  wires:
  bus_creator/1 -> out_port/1  "test_mdl1"
  GearEngag_D_Actl/1 -> bus_creator/1  "GearEngag_D_Actl"
  GearLvr_D_ActlDrv/1 -> bus_creator/2  "GearLvr_D_ActlDrv"
  GearPos_D_Actl/1 -> bus_creator/3  "GearPos_D_Actl"
  GearPos_D_Trg/1 -> bus_creator/4  "GearPos_D_Trg"
  GearPos_No_Cnt/1 -> bus_creator/5  "GearPos_No_Cnt"
  GearPos_No_Cs/1 -> bus_creator/6  "GearPos_No_Cs"
  TrnIgnOffDly_T_Rq/1 -> bus_creator/7  "TrnIgnOffDly_T_Rq"
  TrnPrkSys_D_Actl/1 -> bus_creator/8  "TrnPrkSys_D_Actl"
  TrnRng_D_Rq/1 -> bus_creator/9  "TrnRng_D_Rq"

== system test_mdl1/VehicleCAN/PCM/PowertrainData_2 ==
  ApedPos_Pc_ActlDiag : Constant  Value=0
  EngAirIn_Te_Actl : Constant  Value=0
  EngClnt_Te_ActlDiag : Constant  Value=0
  EngLoad_Pc_CalcDiag : Constant  Value=0
  EngMsgTxt_D_Rq : Constant  Value=0
  GrllShtrPos_B_Falt : Constant  Value=0
  GrllShtrPos_D_Cmd : Constant  Value=0
  IsaOffst_D_Stat : Constant  Value=0
  ObdWarmUp_B_Complt : Constant  Value=0
  SlMde_D_RqDsply : Constant  Value=0
  SlMde_D_Stat : Constant  Value=0
  bus_creator : BusCreator  Inputs=11
  out_port : Outport
  wires:
  bus_creator/1 -> out_port/1  "test_mdl1"
  ApedPos_Pc_ActlDiag/1 -> bus_creator/1  "ApedPos_Pc_ActlDiag"
  EngAirIn_Te_Actl/1 -> bus_creator/2  "EngAirIn_Te_Actl"
  EngClnt_Te_ActlDiag/1 -> bus_creator/3  "EngClnt_Te_ActlDiag"
  EngLoad_Pc_CalcDiag/1 -> bus_creator/4  "EngLoad_Pc_CalcDiag"
  EngMsgTxt_D_Rq/1 -> bus_creator/5  "EngMsgTxt_D_Rq"
  GrllShtrPos_B_Falt/1 -> bus_creator/6  "GrllShtrPos_B_Falt"
  GrllShtrPos_D_Cmd/1 -> bus_creator/7  "GrllShtrPos_D_Cmd"
  IsaOffst_D_Stat/1 -> bus_creator/8  "IsaOffst_D_Stat"
  ObdWarmUp_B_Complt/1 -> bus_creator/9  "ObdWarmUp_B_Complt"
  SlMde_D_RqDsply/1 -> bus_creator/10  "SlMde_D_RqDsply"
  SlMde_D_Stat/1 -> bus_creator/11  "SlMde_D_Stat"

== system test_mdl1/VehicleCAN/PCM/PowertrainData_3 ==
  BattULoChrg_U_Cmd : Constant  Value=0
  ElLoadCtl_D_Rq : Constant  Value=0
  EngMnfld_P_Actl : Constant  Value=0
  FuelPumpPwr_B_Rq : Constant  Value=0
  bus_creator : BusCreator  Inputs=4
  out_port : Outport
  wires:
  bus_creator/1 -> out_port/1  "test_mdl1"
  BattULoChrg_U_Cmd/1 -> bus_creator/1  "BattULoChrg_U_Cmd"
  ElLoadCtl_D_Rq/1 -> bus_creator/2  "ElLoadCtl_D_Rq"
  EngMnfld_P_Actl/1 -> bus_creator/3  "EngMnfld_P_Actl"
  FuelPumpPwr_B_Rq/1 -> bus_creator/4  "FuelPumpPwr_B_Rq"
